simulink model "ksch_5"  (R2014a)
settings: Solver=VariableStepAuto  StartTime=0.0  StopTime=1e3  RelTol=1e-3
libraries: simulink x5, commrfcorlib x1
settings Model: Creator=04sii03  LastModifiedBy=Igor
settings DataIOCC: LimitDataPoints=off  SaveFormat=Dataset
settings OptimizationCC: LifeSpan=auto  SimCompilerOptimization=off
settings DebuggingCC: MergeDetectMultiDrivingBlocksExec=error  SolverPrmCheckMsg=none  FcnCallInpInsideContextMsg=error  FrameProcessingCompatibilityMsg=error  SFUnexpectedBacktrackingDiag=error  SFNoUnconditionalDefaultTransitionDiag=error
settings HardwareCC: ProdBitPerPointer=64  ProdLargestAtomicFloat=Float  ProdIntDivRoundTo=Zero  ProdEndianess=LittleEndian  ProdWordSize=64  ProdHWDeviceType=Intel->x86-64 (Windows64)
settings ModelReferenceCC: PropagateSignalLabelsOutOfModel=on
settings RTWCC: RTWCompilerOptimization=off
settings GRTTargetCC: TargetLangStandard=C99 (ISO)  GeneratePreprocessorConditionals=Use local settings
settings ConfigurationSet: Description=Simscape Multibody

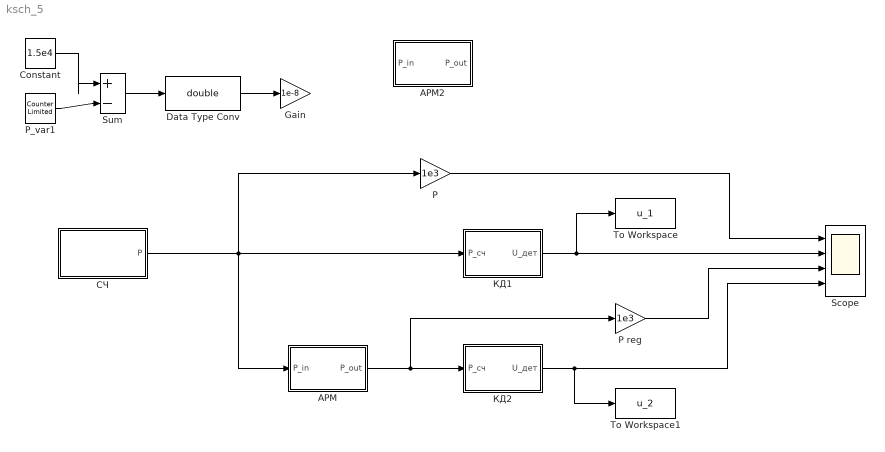
== system ksch_5 ==
  Constant : Constant  Value=1.5e4
  Data Type Conv : DataTypeConversion  OutDataTypeStr=double
  Gain : Gain  Gain=1e-8
  P : Gain  Gain=1e3
  P reg : Gain  Gain=1e3
  P_var1 : simulink/Sources/Counter Limited  uplimit=7  tsamp=-1
  Scope : Scope  NumInputPorts=4
  Sum : Sum  Inputs=|+-
  To Workspace : ToWorkspace  VariableName=u_1  SampleTime=-1
  To Workspace1 : ToWorkspace  VariableName=u_2  SampleTime=-1
  АРМ : Subsystem
  АРМ2 : Subsystem
  КД1 : Subsystem
  КД2 : Subsystem
  СЧ : MATLAB Function  TreatAsAtomicUnit=on
  wires:
  КД1/1(U_дет) -> To Workspace/1, Scope/2
  КД2/1(U_дет) -> To Workspace1/1, Scope/4
  P_var1/1 -> Sum/2
  Data Type Conv/1 -> Gain/1
  Constant/1 -> Sum/1
  Sum/1 -> Data Type Conv/1
  P/1 -> Scope/1
  P reg/1 -> Scope/3
  СЧ/1(P) -> АРМ/1(P_in), P/1, КД1/1(P_сч)
  АРМ/1(P_out) -> КД2/1(P_сч), P reg/1

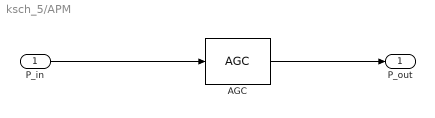
== system ksch_5/АРМ ==
  P_in : Inport
  AGC : commrfcorlib/AGC
  P_out : Outport
  wires:
  P_in/1 -> AGC/1
  AGC/1 -> P_out/1

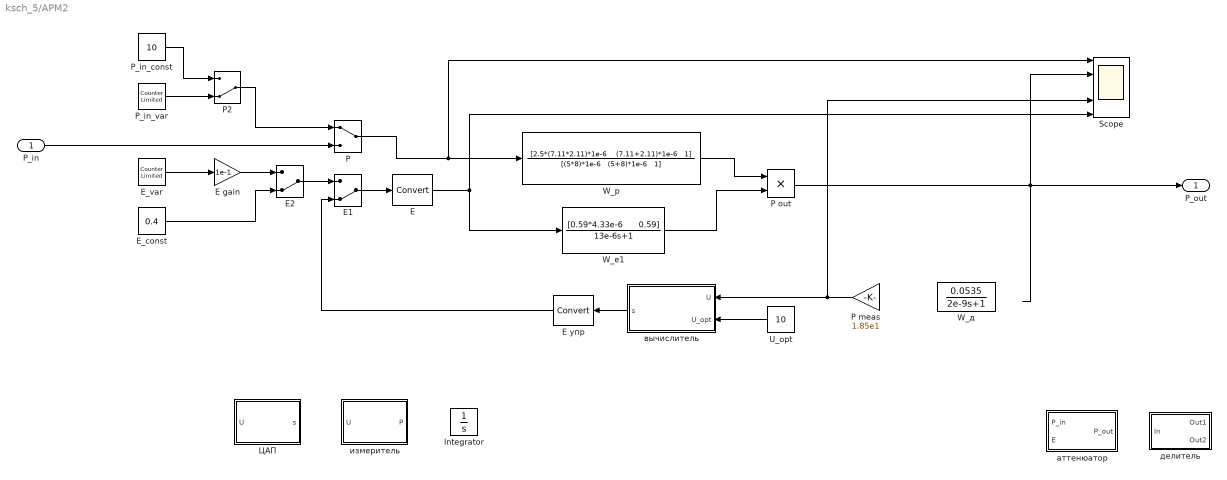
== system ksch_5/АРМ2 ==
  P_in : Inport
  E : DataTypeConversion
  E gain : Gain  Gain=1e-1
  E упр : DataTypeConversion
  E1 : ManualSwitch  CurrentSetting=0
  E2 : ManualSwitch  CurrentSetting=0
  E_const : Constant  Value=0.4
  E_var : simulink/Sources/Counter Limited
  Integrator : Integrator
  P : ManualSwitch
  P meas : Gain  Gain=1.85e1
  P out : Product  Inputs=**
  P2 : ManualSwitch  CurrentSetting=0
  P_in_const : Constant  Value=10
  P_in_var : simulink/Sources/Counter Limited
  Scope : Scope  NumInputPorts=5
  U_opt : Constant  Value=10
  W_e1 : TransferFcn  Numerator="[0.59*4.33e-6      0.59]"  Denominator="[13e-6     1]"
  W_p : TransferFcn  Numerator="[2.5*(7.11*2.11)*1e-6    (7.11+2.11)*1e-6   1]"  Denominator="[(5*8)*1e-6   (5+8)*1e-6   1]"
  W_д : TransferFcn  Numerator="[0      0.0535]"  Denominator="[2e-9    1]"
  ЦАП : MATLAB Function  TreatAsAtomicUnit=on
  аттенюатор : Subsystem
  вычислитель : MATLAB Function  TreatAsAtomicUnit=on
  делитель : Subsystem
  измеритель : MATLAB Function  TreatAsAtomicUnit=on
  P_out : Outport
  wires:
  P2/1 -> P/1
  P_in_const/1 -> P2/1
  P_in_var/1 -> P2/2
  E1/1 -> E/1
  ? -> Scope/3, P meas/1
  вычислитель/1(s) -> E упр/1
  E_var/1 -> E gain/1
  P_in/1 -> P/2
  E2/1 -> E1/1
  E_const/1 -> E2/2
  P out/1 -> Scope/2, P_out/1
  P/1 -> W_p/1, Scope/1
  E/1 -> W_e1/1, Scope/5
  E упр/1 -> E1/2
  U_opt/1 -> вычислитель/2(U_opt)
  P meas/1 -> Scope/4, вычислитель/1(U)
  E gain/1 -> E2/1
  W_p/1 -> P out/1
  W_e1/1 -> P out/2

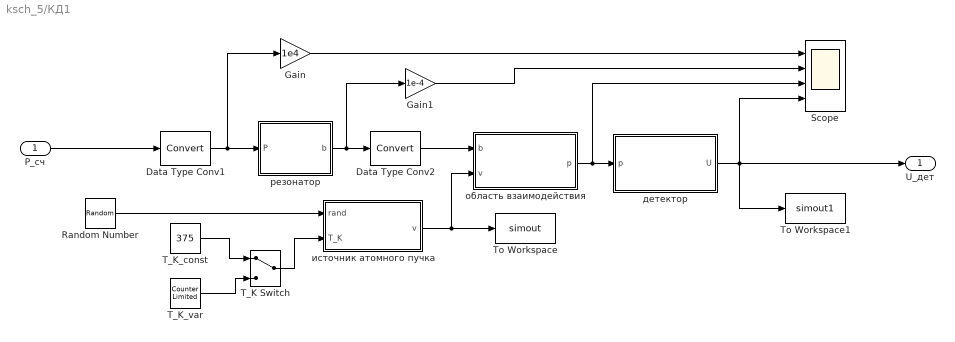
== system ksch_5/КД1 ==
  P_сч : Inport
  Data Type Conv1 : DataTypeConversion
  Data Type Conv2 : DataTypeConversion
  Gain : Gain  Gain=1e4
  Gain1 : Gain  Gain=1e-4
  Random Number : RandomNumber  SampleTime=0.1
  Scope : Scope  NumInputPorts=4
  T_K Switch : ManualSwitch
  T_K_const : Constant  Value=375
  T_K_var : simulink/Sources/Counter Limited  uplimit=7  tsamp=-1
  To Workspace : ToWorkspace  VariableName=simout  SaveFormat=Timeseries  SampleTime=-1
  To Workspace1 : ToWorkspace  VariableName=simout1  SaveFormat=Timeseries  SampleTime=-1
  детектор : MATLAB Function  TreatAsAtomicUnit=on
  источник атомного пучка : MATLAB Function  TreatAsAtomicUnit=on
  область взаимодействия : MATLAB Function  TreatAsAtomicUnit=on
  резонатор : MATLAB Function  TreatAsAtomicUnit=on
  U_дет : Outport
  wires:
  Data Type Conv2/1 -> область взаимодействия/1(b)
  резонатор/1(b) -> Gain1/1, Data Type Conv2/1
  область взаимодействия/1(p) -> Scope/3, детектор/1(p)
  T_K_const/1 -> T_K Switch/1
  P_сч/1 -> Data Type Conv1/1
  Data Type Conv1/1 -> Gain/1, резонатор/1(P)
  детектор/1(U) -> To Workspace1/1, Scope/4, U_дет/1
  T_K Switch/1 -> источник атомного пучка/2(T_K)
  T_K_var/1 -> T_K Switch/2
  Gain/1 -> Scope/1
  Gain1/1 -> Scope/2
  Random Number/1 -> источник атомного пучка/1(rand)
  источник атомного пучка/1(v) -> To Workspace/1, область взаимодействия/2(v)

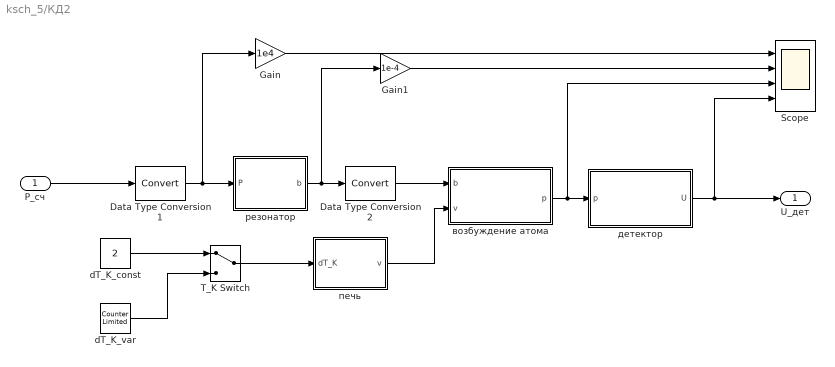
== system ksch_5/КД2 ==
  P_сч : Inport
  Data Type Conversion1 : DataTypeConversion
  Data Type Conversion2 : DataTypeConversion
  Gain : Gain  Gain=1e4
  Gain1 : Gain  Gain=1e-4
  Scope : Scope  NumInputPorts=4
  T_K Switch : ManualSwitch
  dT_K_const : Constant  Value=2
  dT_K_var : simulink/Sources/Counter Limited
  возбуждение атома : MATLAB Function  TreatAsAtomicUnit=on
  детектор : MATLAB Function  TreatAsAtomicUnit=on
  печь : MATLAB Function  TreatAsAtomicUnit=on
  резонатор : MATLAB Function  TreatAsAtomicUnit=on
  U_дет : Outport
  wires:
  Data Type Conversion2/1 -> возбуждение атома/1(b)
  резонатор/1(b) -> Gain1/1, Data Type Conversion2/1
  возбуждение атома/1(p) -> Scope/3, детектор/1(p)
  dT_K_const/1 -> T_K Switch/1
  печь/1(v) -> возбуждение атома/2(v)
  P_сч/1 -> Data Type Conversion1/1
  Data Type Conversion1/1 -> Gain/1, резонатор/1(P)
  детектор/1(U) -> Scope/4, U_дет/1
  T_K Switch/1 -> печь/1(dT_K)
  dT_K_var/1 -> T_K Switch/2
  Gain/1 -> Scope/1
  Gain1/1 -> Scope/2

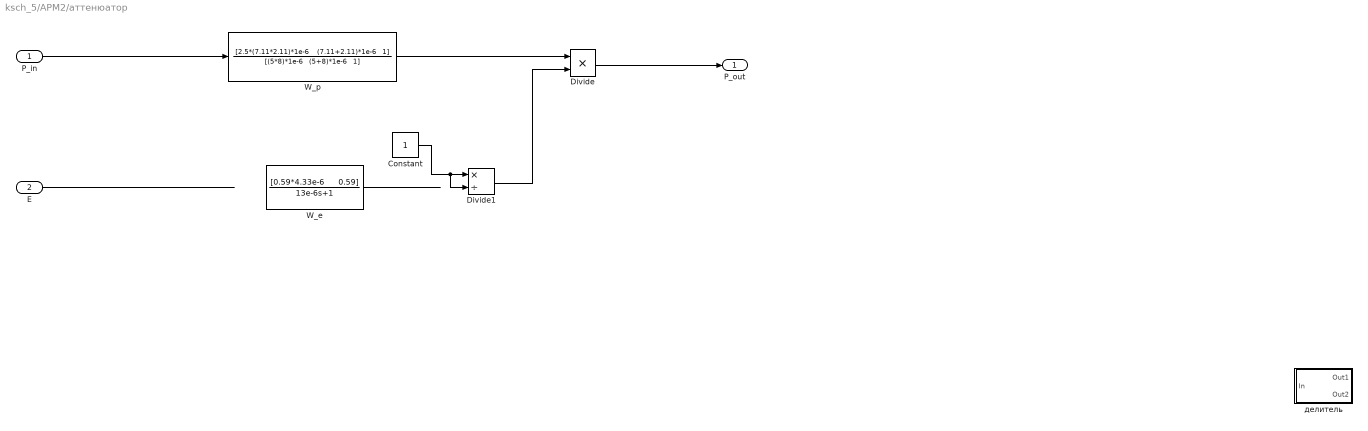
== system ksch_5/АРМ2/аттенюатор ==
  P_in : Inport
  E : Inport  Port=2
  Constant : Constant
  Divide : Product  Inputs=**
  Divide1 : Product  Inputs=*/
  W_e : TransferFcn  Numerator="[0.59*4.33e-6      0.59]"  Denominator="[13e-6     1]"
  W_p : TransferFcn  Numerator="[2.5*(7.11*2.11)*1e-6    (7.11+2.11)*1e-6   1]"  Denominator="[(5*8)*1e-6   (5+8)*1e-6   1]"
  делитель : Subsystem
  P_out : Outport
  wires:
  P_in/1 -> W_p/1
  E/1 -> ?
  Divide/1 -> P_out/1
  W_e/1 -> ?
  W_p/1 -> Divide/1
  Divide1/1 -> Divide/2
  Constant/1 -> Divide1/2, Divide1/1

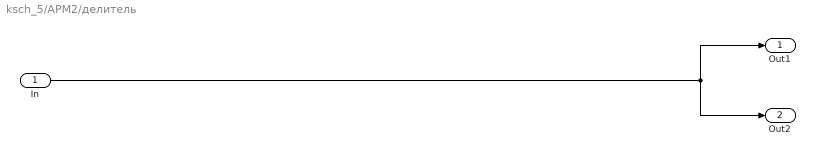
== system ksch_5/АРМ2/делитель ==
  In : Inport
  Out1 : Outport
  Out2 : Outport  Port=2
  wires:
  In/1 -> Out2/1, Out1/1

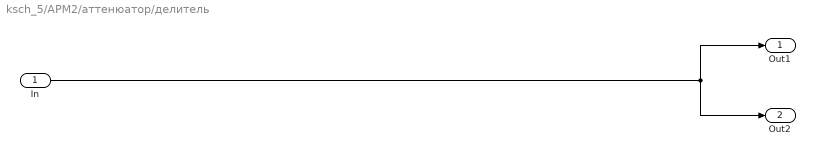
== system ksch_5/АРМ2/аттенюатор/делитель ==
  In : Inport
  Out1 : Outport
  Out2 : Outport  Port=2
  wires:
  In/1 -> Out2/1, Out1/1

== matlab function ksch_5/КД1/возбуждение атома ==
  data: b input; p output; v input
% =========================================================================
% %CESIUM% ATOM EXCITATION
%--------------------------------------------------------------------------
% по Пихтелеву (стр.124)
%--------------------------------------------------------------------------
% p - вероятность атомного перехода
% b - параметр возбуждения
% v - скорость атомов в пучке
% =========================================================================


function p = atom_excitation ( b, v )


%--------------------------------------------------------------------------
% НАЧАЛЬНЫЕ ДАННЫЕ
%--------------------------------------------------------------------------
l = 0.01; % длина области взаимодействия, м
L = 0.15; % длина области пролета, м
f_00 = 9192631770; % частота рабочего атомного перехода (0-0), Гц
v_opt = 216; % оптимальная скорость атомов, м/с
t = l/v;
T = L/v;
dv = 3;
%--------------------------------------------------------------------------


%--------------------------------------------------------------------------
% ВЕРОЯТНОСТЬ РАБОЧЕГО АТОМНОГО ПЕРЕХОДА
%--------------------------------------------------------------------------
f_res = f_00;

w_00 = 2*pi*f_00; % угловая частота рабочего перехода
w_res = 2*pi*f_res; % угловая частота сигнала возбуждения
omega_0 = w_res - w_00; % расстройка угловой частоты сигнала возбуждения
omega = sqrt(b.^2 + omega_0.^2);
ot2 = omega.*(l/(v + rand*dv - dv/2))/2; %f_t(i)
o0T2 = omega_0.*T/2;

p_temp1 = (2*b./omega) .* sin(ot2);
p_temp2 = cos(ot2) .* cos(o0T2);
p_temp3 = (-omega_0./omega) .* sin(ot2) .* sin(o0T2);
p = (p_temp1 .* (p_temp2 - p_temp3)) .^ 2;
%--------------------------------------------------------------------------



end

== matlab function ksch_5/АРМ2/вычислитель ==
  data: U input; s output; U_opt input
% =========================================================================
% ВЫЧИСЛИТЕЛЬ
%--------------------------------------------------------------------------
% s - код управления
% U  - входное напряжение
% U_opt - оптимальное значение напряжения
% =========================================================================


function s = solver ( U, U_opt )


%--------------------------------------------------------------------------
% КОНСТАНТЫ
%--------------------------------------------------------------------------
k = 100; % коэффициент передачи
E_max = 5;


%--------------------------------------------------------------------------
% РАСЧЕТ
%--------------------------------------------------------------------------
s = abs(U-U_opt) / U_opt * E_max * k;% * k;


end

== matlab function ksch_5/КД2/возбуждение атома ==
  data: b input; p output; v input
% =========================================================================
% %CESIUM% ATOM EXCITATION
%--------------------------------------------------------------------------
% по Пихтелеву (стр.124)
%--------------------------------------------------------------------------
% p - вероятность атомного перехода
% b - параметр возбуждения
% v - скорость атомов в пучке
% =========================================================================


function p = atom_excitation ( b, v )


%--------------------------------------------------------------------------
% НАЧАЛЬНЫЕ ДАННЫЕ
%--------------------------------------------------------------------------
l = 0.01; % длина области взаимодействия, м
L = 0.15; % длина области пролета, м
f_00 = 9192631770; % частота рабочего атомного перехода (0-0), Гц
v_opt = 216; % оптимальная скорость атомов, м/с
t = l/v;
T = L/v;
dv = 3;
%--------------------------------------------------------------------------


%--------------------------------------------------------------------------
% ВЕРОЯТНОСТЬ РАБОЧЕГО АТОМНОГО ПЕРЕХОДА
%--------------------------------------------------------------------------
f_res = f_00;

w_00 = 2*pi*f_00; % угловая частота рабочего перехода
w_res = 2*pi*f_res; % угловая частота сигнала возбуждения
omega_0 = w_res - w_00; % расстройка угловой частоты сигнала возбуждения
omega = sqrt(b.^2 + omega_0.^2);
ot2 = omega.*(l/(v_opt + rand*dv - dv/2))/2; %f_t(i)
o0T2 = omega_0.*T/2;

p_temp1 = (2*b./omega) .* sin(ot2);
p_temp2 = cos(ot2) .* cos(o0T2);
p_temp3 = (-omega_0./omega) .* sin(ot2) .* sin(o0T2);
p = (p_temp1 .* (p_temp2 - p_temp3)) .^ 2;
%--------------------------------------------------------------------------



end

== matlab function ksch_5/КД2/детектор ==
  data: p input; U output
% =========================================================================
% DETECTOR
%--------------------------------------------------------------------------
% u - выходное напряжение детектора
% p - вероятность атомного перехода
% =========================================================================


function U = detector ( p )


%--------------------------------------------------------------------------
% НАЧАЛЬНЫЕ ДАННЫЕ
%--------------------------------------------------------------------------
% l = 0.01; % длина области взаимодействия, м
%--------------------------------------------------------------------------


%--------------------------------------------------------------------------
% РАСЧЕТ
%--------------------------------------------------------------------------
U = p;

%--------------------------------------------------------------------------



end

== matlab function ksch_5/КД2/печь ==
  data: dT_K input; v output
% =========================================================================
% АТОМНАЯ ПЕЧЬ
%--------------------------------------------------------------------------
% v - наиболее вероятная скорость
% dT_K - СКО рабочей температуры печи
% =========================================================================


function v = source ( dT_K )


%--------------------------------------------------------------------------
% ПОСТОЯННЫЕ
%--------------------------------------------------------------------------
k = 1.380649e-23; % постоянная Больцмана
T_K_opt = 375; % рабочая температура, К
m = 132.90545193324 * 1.660539066605e-27; % масса атома (перевод а.е.м. в кг)


%--------------------------------------------------------------------------
% РАСЧЕТ
%--------------------------------------------------------------------------
T_K = T_K_opt + dT_K;
v = sqrt (2*k*T_K/m);

% for (i = 1:5000)
%     p_temp1 = 1 / (sqrt(pi*v));
%     p_temp2 = exp ( (-1) * (i/v)^2 );
%     p(i) = p_temp1 * p_temp2;
% end;
% 
% figure(1); hold on; grid on;
% stairs(p);

end

== matlab function ksch_5/КД1/детектор ==
  data: p input; U output
% =========================================================================
% DETECTOR
%--------------------------------------------------------------------------
% u - выходное напряжение детектора
% p - вероятность атомного перехода
% =========================================================================


function U = detector ( p )


%--------------------------------------------------------------------------
% НАЧАЛЬНЫЕ ДАННЫЕ
%--------------------------------------------------------------------------
% l = 0.01; % длина области взаимодействия, м
%--------------------------------------------------------------------------


%--------------------------------------------------------------------------
% РАСЧЕТ
%--------------------------------------------------------------------------
U = p;

%--------------------------------------------------------------------------



end

== matlab function ksch_5/КД1/печь ==
  data: dT_K input; v output
% =========================================================================
% АТОМНАЯ ПЕЧЬ
%--------------------------------------------------------------------------
% v - наиболее вероятная скорость
% dT_K - СКО рабочей температуры печи
% =========================================================================


function v = source ( dT_K )


%--------------------------------------------------------------------------
% ПОСТОЯННЫЕ
%--------------------------------------------------------------------------
k = 1.380649e-23; % постоянная Больцмана
T_K_opt = 375; % рабочая температура, К
m = 132.90545193324 * 1.660539066605e-27; % масса атома (перевод а.е.м. в кг)
n_1 = 1;
n_2 = 2;
n_3 = 3;
C_n_1 = 2;
C_n_2 = 4/sqrt(pi);
C_n_3 = 2;


%--------------------------------------------------------------------------
% РАСЧЕТ
%--------------------------------------------------------------------------
T_K = T_K_opt + dT_K;
v = sqrt (2*k*T_K/m);


for i = 1:1500
%     fv_1(i) = (C_n_1/v) * (v/v_v(i))^(n_1+2) * exp( -1*(v^2) / (v_v(i)^2) );
    fv_2 = (C_n_2/v) * (v/i)^(n_2+2) * exp( -1*(v^2) / (i^2) );
%     fv_3(i) = (C_n_3/v) * (v/v_v(i))^(n_3+2) * exp( -1*(v^2) / (v_v(i)^2) );
end


xCDF = i;
yCDF = cumsum(fv_2)/sum(fv_2);   %Generate CDF

x1 = rand(1,1);               %Generate uniform random variable
[yCDF, index] = unique(yCDF);
v = interp1(yCDF, xCDF(index), x1);     %Inverse transform

% for (i = 1:5000)
%     p_temp1 = 1 / (sqrt(pi*v));
%     p_temp2 = exp ( (-1) * (i/v)^2 );
%     p(i) = p_temp1 * p_temp2;
% end;
% 
% figure(1); hold on; grid on;
% stairs(p);

end

== matlab function ksch_5/КД1/резонатор ==
  data: P input; b output
% =========================================================================
% АТОМНАЯ ПЕЧЬ
%--------------------------------------------------------------------------
% b - параметр возбуждения
% U - входное напряжение
% dU - СКО напряжения U
% =========================================================================


function b = cavity ( P ) %, dU )


%--------------------------------------------------------------------------
% КОНСТАНТЫ
%--------------------------------------------------------------------------
h = 6.62607015e-34; % постоянная Планка
g_j = 2; % множитель (g-фактор) Ланде
mu_0 = 1.25663706212e-6; %927.400968e-26; % магнитная проницаемость вакуума
mu_b = 5.05e-24; % ядерный магнетон Бора
a_res = 0.023; % ширина поперечного сечения волноводного резонатора a, м
b_res = 0.01; % высота поперечного сечения волноводного резонатора b, м
Q_res = 1e3; % добротность резонатора
Z_0 = 376.73; % волновое сопротивление вакуума (в резонаторе), Ом
S = a_res * b_res; % площадь поперечного сечения волноводного резонатора, м^2


%--------------------------------------------------------------------------
% РАСЧЕТ
%--------------------------------------------------------------------------
P_res = P * Q_res; % мощность в резонаторе
H = sqrt ( (2*P_res) / (Z_0*S) );
B = H * mu_0;
b = (g_j*mu_b*B)/(h);

end

== matlab function ksch_5/КД2/резонатор ==
  data: P input; b output
% =========================================================================
% АТОМНАЯ ПЕЧЬ
%--------------------------------------------------------------------------
% b - параметр возбуждения
% U - входное напряжение
% dU - СКО напряжения U
% =========================================================================


function b = cavity ( P ) %, dU )


%--------------------------------------------------------------------------
% КОНСТАНТЫ
%--------------------------------------------------------------------------
h = 6.62607015e-34; % постоянная Планка
g_j = 2; % множитель (g-фактор) Ланде
mu_0 = 1.25663706212e-6; %927.400968e-26; % магнитная проницаемость вакуума
mu_b = 5.05e-24; % ядерный магнетон Бора
a_res = 0.023; % ширина поперечного сечения волноводного резонатора a, м
b_res = 0.01; % высота поперечного сечения волноводного резонатора b, м
Q_res = 1e3; % добротность резонатора
Z_0 = 376.73; % волновое сопротивление вакуума (в резонаторе), Ом
S = a_res * b_res; % площадь поперечного сечения волноводного резонатора, м^2


%--------------------------------------------------------------------------
% РАСЧЕТ
%--------------------------------------------------------------------------
P_res = P * Q_res; % мощность в резонаторе
H = sqrt ( (2*P_res) / (Z_0*S) );
B = H * mu_0;
b = (g_j*mu_b*B)/(h);

end

== matlab function ksch_5/СЧ ==
  data: P output
% =========================================================================
% SYNTHESIZER
%--------------------------------------------------------------------------
% u - напряжение выходного сигнала синтезатора
% =========================================================================


function P = synthesizer ( )


%--------------------------------------------------------------------------
% НАЧАЛЬНЫЕ ДАННЫЕ
%--------------------------------------------------------------------------
% l = 0.01; % длина области взаимодействия, м
%--------------------------------------------------------------------------


%--------------------------------------------------------------------------
% РАСЧЕТ
%--------------------------------------------------------------------------
P = 0,000123;

%--------------------------------------------------------------------------



end

== matlab function ksch_5/АРМ2/измеритель ==
  data: P input; U output
% =========================================================================
% ИЗМЕРИТЕЛЬ
%--------------------------------------------------------------------------
% P - входная мощность
% U  - выходное напряжение
% =========================================================================


function U = powermeter ( P )


%--------------------------------------------------------------------------
% КОНСТАНТЫ
%--------------------------------------------------------------------------
k2 = 0.5;%0.0535;%2.22e-2; % коэффициент передачи
T1 = 1;%2e-6;


%--------------------------------------------------------------------------
% РАСЧЕТ
%--------------------------------------------------------------------------
W_d = k2 / (T1*P+1);
U = W_d;


end

== matlab function ksch_5/АРМ2/ЦАП ==
  data: s input; U output
% =========================================================================
% ЦИФРО-АНАЛОГОВЫЙ ПРЕОБРАЗОВАТЕЛЬ
%--------------------------------------------------------------------------
% s - код управления
% U  - выходное напряжение
% =========================================================================


function U = dac ( s )


%--------------------------------------------------------------------------
% КОНСТАНТЫ
%--------------------------------------------------------------------------
k = 0.023; % коэффициент передачи


%--------------------------------------------------------------------------
% РАСЧЕТ
%--------------------------------------------------------------------------
U = s;


end

== matlab function ksch_5/КД1/источник атомного пучка ==
  data: rand input; T_K input; v output
function v = source ( rand, T_K )


%--------------------------------------------------------------------------
% ПОСТОЯННЫЕ
%--------------------------------------------------------------------------
k = 1.380649e-23; % постоянная Больцмана
T_K_opt = 375; % рабочая температура, К
m = 132.90545193324 * 1.660539066605e-27; % масса атома (перевод а.е.м. в кг)
L = 0.15;
l = 0.01;
n_1 = 1;
n_2 = 2;
n_3 = 3;
C_n_1 = 2;
C_n_2 = 4/sqrt(pi);
C_n_3 = 2;


%--------------------------------------------------------------------------
% РАСЧЕТ
%--------------------------------------------------------------------------
T_K = T_K_opt; %+ dT_K;
v = sqrt (2*k*T_K/m);
% dv = 1;
t_0 = l/v;


for i = 1:3000
    v_v(i) = i;% - 750;
%     v_x(i) = v_v(i) + v;
    
    
    t(i) = (i) * 1e-7;
%     t_x(i) = t(i);
    
    
    %----------------------------------------------------------------------
    % Риле (стр. 152)
    %----------------------------------------------------------------------
%     p_temp1(i) = 1 / (sqrt(pi)*v);
%     p_temp2(i) = exp ( (-1) * (v_v(i)/v)^2 );
%     p(i) = p_temp1(i) * p_temp2(i);


    %----------------------------------------------------------------------
    % Xie "Linewidth locking method" & "Research on Main Kinds of Frequency
    % Biases"
    %----------------------------------------------------------------------
    ft_exp(i) = exp( -1*(t_0^2) / (t(i)^2) );
    ft_n1(i) = (t_0/t(i))^(n_1+2);
    ft_n2(i) = (t_0/t(i))^(n_2+2);
    ft_n3(i) = (t_0/t(i))^(n_3+2);
    fv_1(i) = (C_n_1/t_0) * ft_n1(i) * ft_exp(i);
    fv_2(i) = (C_n_2/t_0) * ft_n2(i) * ft_exp(i);
    fv_3(i) = (C_n_3/t_0) * ft_n3(i) * ft_exp(i);

%     fv_1(i) = 1 / (sqrt(pi*v)) * exp( (-1) * ((v/v_v(i))^2) );
%     fv_1(i) = (C_n_1/v) * (v/v_v(i))^(n_1+2) * exp( (-1) * ((v/v_v(i))^2) );
%     fv_2(i) = (C_n_2/v) * (v/v_v(i))^(n_2+2) * exp( (-1) * ((v/v_v(i))^2) );
%     fv_3(i) = (C_n_3/v) * (v/v_v(i))^(n_3+2) * exp( (-1) * ((v/v_v(i))^2) );

    % fv_1_sum = sum (fv_1)
    % fv_2_sum = sum (fv_2)
    % fv_3_sum = sum (fv_3)


end


xCDF = t;%v_v;

% Generate CDF
yCDF1 = cumsum(fv_1)/sum(fv_1);
yCDF2 = cumsum(fv_2)/sum(fv_2);
yCDF3 = cumsum(fv_3)/sum(fv_3);

% Generate uniform random variable
x1_1 = rand(1e5,1);

[yCDF1, index] = unique(yCDF1);
[yCDF2, index] = unique(yCDF2);
[yCDF3, index] = unique(yCDF3);

% Inverse transform
x1 = interp1(yCDF1, xCDF(index), x1_1);
x2 = interp1(yCDF2, xCDF(index), x1_1);
x3 = interp1(yCDF3, xCDF(index), x1_1);

end
